simulink model "OperationalSpaceSpaceGravityCompensation"  (R2020b)
settings: Solver=VariableStepAuto  StartTime=0.0  StopTime=20  RelTol=1e-3
values from neighbouring files (symbols this model uses):
  KD = diag([  35   45   15    1     0   0])    [parameters.m]
  KP = diag([ 250  350  100   50     1   1])    [parameters.m]
libraries: vrlib x1
settings Model: Creator=Edoardo  LastModifiedBy=Edoardo

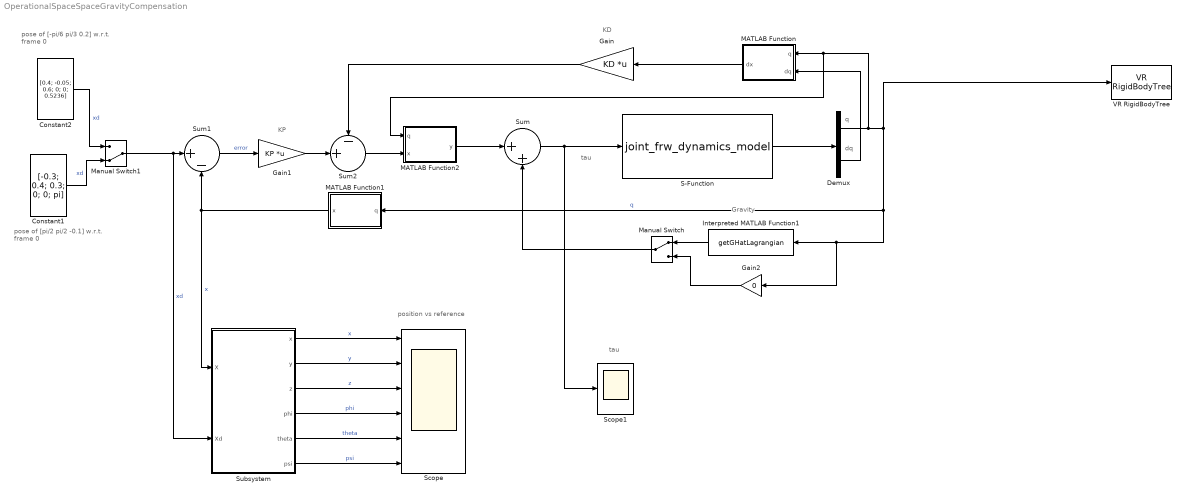
== system OperationalSpaceSpaceGravityCompensation ==
  note: tau
  note: Gravity
  note: tau
  note: KP
  note: KD
  note: dq
  note: q
  note: position vs reference
  note: pose of [pi/2 pi/2 -0.1]
      | w.r.t. frame 0
  note: pose of [-pi/6 pi/3 0.2]
      | w.r.t. frame 0
  Constant1 : Constant  Value=[-0.3; 0.4; 0.3; 0; 0; pi]  VectorParams1D=off
  Constant2 : Constant  Value=[0.4; -0.05; 0.6; 0; 0; 0.5236]  VectorParams1D=off
  Demux : Demux  Outputs=2
  Gain : Gain  Gain=KD  Multiplication=Matrix(K*u) (u vector)
  Gain1 : Gain  Gain=KP  Multiplication=Matrix(K*u) (u vector)
  Gain2 : Gain  Gain=0
  Interpreted MATLAB Function1 : MATLABFcn  MATLABFcn=getGHatLagrangian
  MATLAB Function : MATLAB Function  TreatAsAtomicUnit=on
  MATLAB Function1 : MATLAB Function  TreatAsAtomicUnit=on
  MATLAB Function2 : MATLAB Function  TreatAsAtomicUnit=on
  Manual Switch : ManualSwitch
  Manual Switch1 : ManualSwitch  CurrentSetting=0
  S-Function : S-Function  FunctionName=joint_frw_dynamics_model  Parameters=myRobot  SFunctionDeploymentMode=off  EnableBusSupport=off
  Scope : Scope  NumInputPorts=6
  Scope1 : Scope
  Subsystem : Subsystem
  Sum : Sum  Inputs=|++
  Sum1 : Sum  Inputs=|+-
  Sum2 : Sum  Inputs=-+|
  VR RigidBodyTree : vrlib/VR RigidBodyTree  RBT=robot  useRBT=on  Ts=-1  ForceViewerOpen=on
      settings: SourceProductBaseCode=SL
  wires:
  S-Function/1 -> Demux/1
  Sum/1 -> Scope1/1, S-Function/1
  Gain/1 -> Sum2/1
  Sum1/1 -> Gain1/1  "error"
  Demux/1 -> MATLAB Function/1(q), MATLAB Function2/1(q), VR RigidBodyTree/1, Gain2/1, Interpreted MATLAB Function1/1, MATLAB Function1/1(q)  "q"
  Gain1/1 -> Sum2/2
  Manual Switch1/1 -> Subsystem/2(Xd), Sum1/1  "xd"
  Gain2/1 -> Manual Switch/2
  Manual Switch/1 -> Sum/2
  Interpreted MATLAB Function1/1 -> Manual Switch/1
  Demux/2 -> MATLAB Function/2(dq)
  MATLAB Function/1(dx) -> Gain/1
  MATLAB Function1/1(x) -> Subsystem/1(X), Sum1/2  "x"
  Sum2/1 -> MATLAB Function2/2(x)
  MATLAB Function2/1(y) -> Sum/1
  Constant1/1 -> Manual Switch1/2  "xd"
  Constant2/1 -> Manual Switch1/1  "xd"
  Subsystem/1(x) -> Scope/1  "x"
  Subsystem/2(y) -> Scope/2  "y"
  Subsystem/3(z) -> Scope/3  "z"
  Subsystem/4(phi) -> Scope/4  "phi"
  Subsystem/5(theta) -> Scope/5  "theta"
  Subsystem/6(psi) -> Scope/6  "psi"

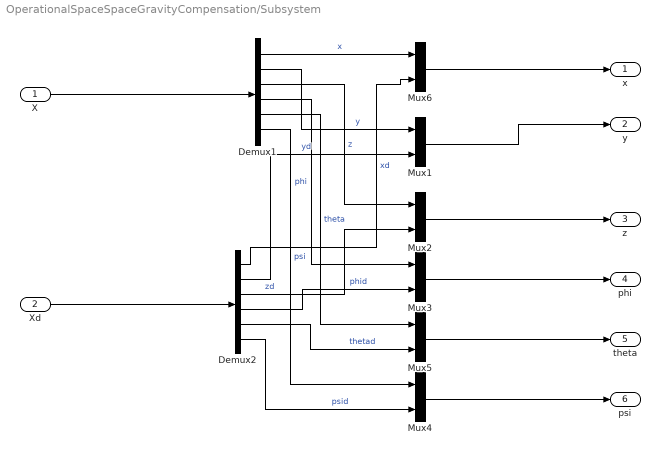
== system OperationalSpaceSpaceGravityCompensation/Subsystem ==
  X : Inport
  Xd : Inport  Port=2
  Demux1 : Demux  Outputs=6
  Demux2 : Demux  Outputs=6
  Mux{1..6} (6 alike) : Mux  Inputs=2
  x : Outport
  y : Outport  Port=2
  z : Outport  Port=3
  phi : Outport  Port=4
  theta : Outport  Port=5
  psi : Outport  Port=6
  wires:
  Demux1/3 -> Mux2/1  "z"
  Demux1/4 -> Mux3/1  "phi"
  Demux2/3 -> Mux2/2  "zd"
  Mux2/1 -> z/1
  Demux2/1 -> Mux6/2  "xd"
  Demux1/5 -> Mux5/1  "theta"
  Mux1/1 -> y/1
  Demux1/6 -> Mux4/1  "psi"
  Demux1/1 -> Mux6/1  "x"
  Demux2/5 -> Mux5/2  "thetad"
  Demux2/6 -> Mux4/2  "psid"
  Demux1/2 -> Mux1/1  "y"
  Demux2/4 -> Mux3/2  "phid"
  Demux2/2 -> Mux1/2  "yd"
  Xd/1 -> Demux2/1
  X/1 -> Demux1/1
  Mux3/1 -> phi/1
  Mux5/1 -> theta/1
  Mux4/1 -> psi/1
  Mux6/1 -> x/1

== matlab function OperationalSpaceSpaceGravityCompensation/MATLAB Function ==
  data: q input size=3; dx output size=6; dq input size=3
function dx = JA(q,dq)

dx = getAnalyticalJacobian(q)*dq;

== matlab function OperationalSpaceSpaceGravityCompensation/MATLAB Function2 ==
  data: q input size=3; y output size=3; x input
function y = JAT(q,x)

y = getAnalyticalJacobian(q)'*x;

== matlab function OperationalSpaceSpaceGravityCompensation/MATLAB Function1 ==
  data: q input size=3; x output size=6
function x = K(q)

K = getDirectKinematics(q);

pos = K(1:3, 4);
rotm = K(1:3,1:3); 
ori = rotm2eul(rotm, 'ZYZ')';

x = [pos; ori];
